simulink model "lab2_ex5"  (Simulink 6.0)
settings: Solver=ode45  StartTime=0.0  StopTime=10.0  RelTol=1e-3
undefined symbols (not defined in the file): k
settings Model: LastModifiedBy=student

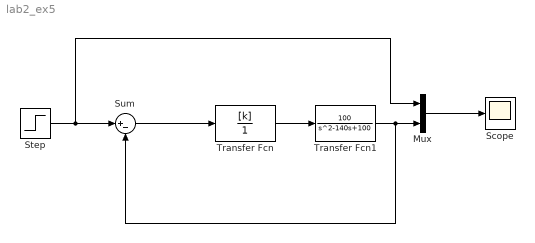
== system lab2_ex5 ==
  Mux : Mux  Inputs=2
  Scope : Scope
  Step : Step  SampleTime=0  ZeroCross=off
  Sum : Sum  Inputs=|+-
  Transfer Fcn : TransferFcn  Numerator=[k]  Denominator=[1]
  Transfer Fcn1 : TransferFcn  Numerator=[100]  Denominator=[1 -140 100]
  wires:
  Mux/1 -> Scope/1
  Transfer Fcn/1 -> Transfer Fcn1/1
  Transfer Fcn1/1 -> Mux/2, Sum/2
  Sum/1 -> Transfer Fcn/1
  Step/1 -> Sum/1, Mux/1
